simulink model "IEEE_30_Bus_System"  (R2021a)
settings: Solver=FixedStepDiscrete  StartTime=0.0  StopTime=0.5  FixedStep=50e-6  RelTol=1e-3
undefined symbols (not defined in the file): Angle, Magnitude, V_890, Vnom1
libraries: spsThreePhasePISectionLineLib x37, spsThreePhaseVIMeasurementLib x30, spsLoadFlowBusLib x30, spsThreePhaseSeriesRLCLoadLib x21, spsThreePhaseSourceLib x6, spsThreePhaseTransformerTwoWindingsLib x4, spspowerguiLib x1
(part 1 of 2)
settings Model: Creator=liyifu  LastModifiedBy=shiyu
settings SolverCC: AlgebraicLoopSolver=TrustRegion
settings DataIOCC: ReturnWorkspaceOutputs=off
settings DebuggingCC: SFMachineParentedDataDiag=warning  ArithmeticOperatorsInVariantConditions=warning
settings SFSimCC: SimUseLocalCustomCode=off  CustomCodeUndefinedFunction=UseInterfaceOnly
settings RTWCC: RTWUseLocalCustomCode=off

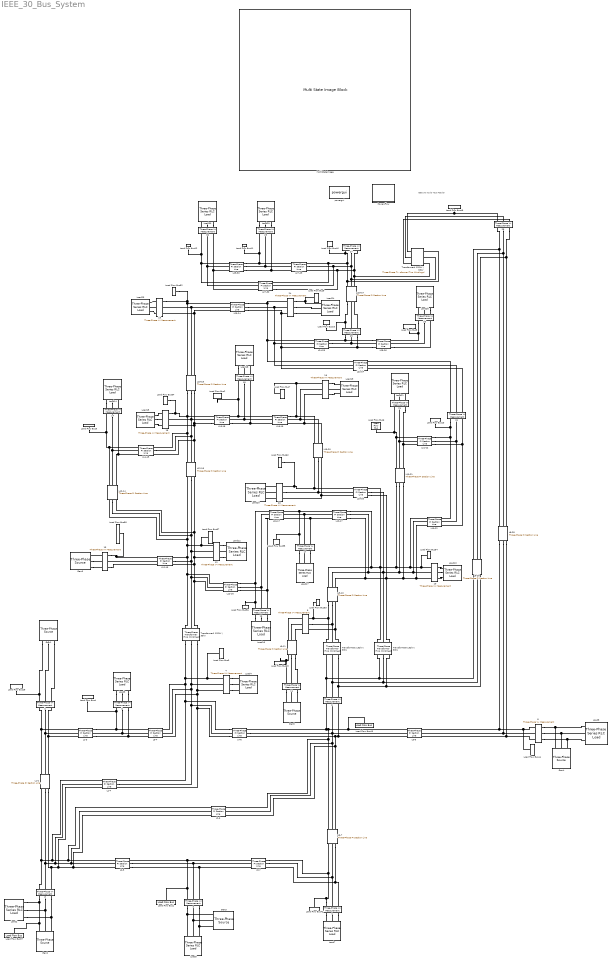
== system IEEE_30_Bus_System ==
  note: IEEE 30 Node Test Feeder
  1 : spsThreePhaseVIMeasurementLib/Three-Phase V-I Measurement  VoltageMeasurement=phase-to-ground  SetLabelV=on  LabelV=Vabc_1  Vpu=on  VpuLL=off  CurrentMeasurement=yes  SetLabelI=on  LabelI=Iabc_1  Ipu=on  Pbase=100e6  Vbase=132e3  OutputType=Magnitude-Angle  PhasorSimulation=off  PSBequivalent=0
  10 : spsThreePhaseVIMeasurementLib/Three-Phase V-I Measurement  VoltageMeasurement=phase-to-ground  SetLabelV=on  LabelV=Vabc_10  Vpu=on  VpuLL=off  CurrentMeasurement=yes  SetLabelI=on  LabelI=Iabc_10  Ipu=on  Pbase=100e6  Vbase=33e3  OutputType=Magnitude-Angle  PhasorSimulation=off  PSBequivalent=0
  11 : spsThreePhaseVIMeasurementLib/Three-Phase V-I Measurement  VoltageMeasurement=phase-to-ground  SetLabelV=on  LabelV=Vabc_11  Vpu=on  VpuLL=off  CurrentMeasurement=yes  SetLabelI=on  LabelI=Iabc_11  Ipu=on  Pbase=100e6  Vbase=33e3  OutputType=Magnitude-Angle  PhasorSimulation=off  PSBequivalent=0
  12 : spsThreePhaseVIMeasurementLib/Three-Phase V-I Measurement  VoltageMeasurement=phase-to-ground  SetLabelV=on  LabelV=Vabc_12  Vpu=on  VpuLL=off  CurrentMeasurement=yes  SetLabelI=on  LabelI=Iabc_12  Ipu=on  Pbase=100e6  Vbase=33e3  OutputType=Magnitude-Angle  PhasorSimulation=off  PSBequivalent=0
  13 : spsThreePhaseVIMeasurementLib/Three-Phase V-I Measurement  VoltageMeasurement=phase-to-ground  SetLabelV=on  LabelV=Vabc_13  Vpu=on  VpuLL=off  CurrentMeasurement=yes  SetLabelI=on  LabelI=Iabc_13  Ipu=on  Pbase=100e6  Vbase=33e3  OutputType=Magnitude-Angle  PhasorSimulation=off  PSBequivalent=0
  14 : spsThreePhaseVIMeasurementLib/Three-Phase V-I Measurement  VoltageMeasurement=phase-to-ground  SetLabelV=on  LabelV=Vabc_14  Vpu=on  VpuLL=off  CurrentMeasurement=yes  SetLabelI=on  LabelI=Iabc_14  Ipu=on  Pbase=100e6  Vbase=33e3  OutputType=Magnitude-Angle  PhasorSimulation=off  PSBequivalent=0
  15 : spsThreePhaseVIMeasurementLib/Three-Phase V-I Measurement  VoltageMeasurement=phase-to-ground  SetLabelV=on  LabelV=Vabc_15  Vpu=on  VpuLL=off  CurrentMeasurement=yes  SetLabelI=on  LabelI=Iabc_15  Ipu=on  Pbase=100e6  Vbase=33e3  OutputType=Magnitude-Angle  PhasorSimulation=off  PSBequivalent=0
  16 : spsThreePhaseVIMeasurementLib/Three-Phase V-I Measurement  VoltageMeasurement=phase-to-ground  SetLabelV=on  LabelV=Vabc_16  Vpu=on  VpuLL=off  CurrentMeasurement=yes  SetLabelI=on  LabelI=Iabc_16  Ipu=on  Pbase=100e6  Vbase=33e3  OutputType=Magnitude-Angle  PhasorSimulation=off  PSBequivalent=0
  17 : spsThreePhaseVIMeasurementLib/Three-Phase V-I Measurement  VoltageMeasurement=phase-to-ground  SetLabelV=on  LabelV=Vabc_17  Vpu=on  VpuLL=off  CurrentMeasurement=yes  SetLabelI=on  LabelI=Iabc_17  Ipu=on  Pbase=100e6  Vbase=33e3  OutputType=Magnitude-Angle  PhasorSimulation=off  PSBequivalent=0
  18 : spsThreePhaseVIMeasurementLib/Three-Phase V-I Measurement  VoltageMeasurement=phase-to-ground  SetLabelV=on  LabelV=Vabc_18  Vpu=on  VpuLL=off  CurrentMeasurement=yes  SetLabelI=on  LabelI=Iabc_18  Ipu=on  Pbase=100e6  Vbase=33e3  OutputType=Magnitude-Angle  PhasorSimulation=off  PSBequivalent=0
  19 : spsThreePhaseVIMeasurementLib/Three-Phase V-I Measurement  VoltageMeasurement=phase-to-ground  SetLabelV=on  LabelV=Vabc_19  Vpu=on  VpuLL=off  CurrentMeasurement=yes  SetLabelI=on  LabelI=Iabc_19  Ipu=on  Pbase=100e6  Vbase=33e3  OutputType=Magnitude-Angle  PhasorSimulation=off  PSBequivalent=0
  2 : spsThreePhaseVIMeasurementLib/Three-Phase V-I Measurement  VoltageMeasurement=phase-to-ground  SetLabelV=on  LabelV=Vabc_2  Vpu=on  VpuLL=off  CurrentMeasurement=yes  SetLabelI=on  LabelI=Iabc_2  Ipu=on  Pbase=100e6  Vbase=132e3  OutputType=Magnitude-Angle  PhasorSimulation=off  PSBequivalent=0
  20 : spsThreePhaseVIMeasurementLib/Three-Phase V-I Measurement  VoltageMeasurement=phase-to-ground  SetLabelV=on  LabelV=Vabc_20  Vpu=on  VpuLL=off  CurrentMeasurement=yes  SetLabelI=on  LabelI=Iabc_20  Ipu=on  Pbase=100e6  Vbase=33e3  OutputType=Magnitude-Angle  PhasorSimulation=off  PSBequivalent=0
  21 : spsThreePhaseVIMeasurementLib/Three-Phase V-I Measurement  VoltageMeasurement=phase-to-ground  SetLabelV=on  LabelV=Vabc_21  Vpu=on  VpuLL=off  CurrentMeasurement=yes  SetLabelI=on  LabelI=Iabc_21  Ipu=on  Pbase=100e6  Vbase=33e3  OutputType=Magnitude-Angle  PhasorSimulation=off  PSBequivalent=0
  22 : spsThreePhaseVIMeasurementLib/Three-Phase V-I Measurement  VoltageMeasurement=phase-to-ground  SetLabelV=on  LabelV=Vabc_22  Vpu=on  VpuLL=off  CurrentMeasurement=yes  SetLabelI=on  LabelI=Iabc_22  Ipu=on  Pbase=100e6  Vbase=33e3  OutputType=Magnitude-Angle  PhasorSimulation=off  PSBequivalent=0
  23 : spsThreePhaseVIMeasurementLib/Three-Phase V-I Measurement  VoltageMeasurement=phase-to-ground  SetLabelV=on  LabelV=Vabc_23  Vpu=on  VpuLL=off  CurrentMeasurement=yes  SetLabelI=on  LabelI=Iabc_23  Ipu=on  Pbase=100e6  Vbase=33e3  OutputType=Magnitude-Angle  PhasorSimulation=off  PSBequivalent=0
  24 : spsThreePhaseVIMeasurementLib/Three-Phase V-I Measurement  VoltageMeasurement=phase-to-ground  SetLabelV=on  LabelV=Vabc_24  Vpu=on  VpuLL=off  CurrentMeasurement=yes  SetLabelI=on  LabelI=Iabc_24  Ipu=on  Pbase=100e6  Vbase=33e3  OutputType=Magnitude-Angle  PhasorSimulation=off  PSBequivalent=0
  25 : spsThreePhaseVIMeasurementLib/Three-Phase V-I Measurement  VoltageMeasurement=phase-to-ground  SetLabelV=on  LabelV=Vabc_25  Vpu=on  VpuLL=off  CurrentMeasurement=yes  SetLabelI=on  LabelI=Iabc_25  Ipu=on  Pbase=100e6  Vbase=33e3  OutputType=Magnitude-Angle  PhasorSimulation=off  PSBequivalent=0
  26 : spsThreePhaseVIMeasurementLib/Three-Phase V-I Measurement  VoltageMeasurement=phase-to-ground  SetLabelV=on  LabelV=Vabc_26  Vpu=on  VpuLL=off  CurrentMeasurement=yes  SetLabelI=on  LabelI=Iabc_26  Ipu=on  Pbase=100e6  Vbase=33e3  OutputType=Magnitude-Angle  PhasorSimulation=off  PSBequivalent=0
  27 : spsThreePhaseVIMeasurementLib/Three-Phase V-I Measurement  VoltageMeasurement=phase-to-ground  SetLabelV=on  LabelV=Vabc_27  Vpu=off  VpuLL=off  CurrentMeasurement=no  SetLabelI=on  LabelI=Iabc_27  Ipu=on  Pbase=100e6  Vbase=33e3  OutputType=Magnitude-Angle  PhasorSimulation=off  PSBequivalent=0
  28 : spsThreePhaseVIMeasurementLib/Three-Phase V-I Measurement  VoltageMeasurement=phase-to-ground  SetLabelV=on  LabelV=Vabc_28  Vpu=on  VpuLL=off  CurrentMeasurement=yes  SetLabelI=on  LabelI=Iabc_28  Ipu=on  Pbase=100e6  Vbase=132e3  OutputType=Magnitude-Angle  PhasorSimulation=off  PSBequivalent=0
  29 : spsThreePhaseVIMeasurementLib/Three-Phase V-I Measurement  VoltageMeasurement=phase-to-ground  SetLabelV=on  LabelV=Vabc_29  Vpu=on  VpuLL=off  CurrentMeasurement=yes  SetLabelI=on  LabelI=Iabc_29  Ipu=on  Pbase=100e6  Vbase=33e3  OutputType=Magnitude-Angle  PhasorSimulation=off  PSBequivalent=0
  3 : spsThreePhaseVIMeasurementLib/Three-Phase V-I Measurement  VoltageMeasurement=phase-to-ground  SetLabelV=on  LabelV=Vabc_3  Vpu=on  VpuLL=off  CurrentMeasurement=yes  SetLabelI=on  LabelI=Iabc_3  Ipu=on  Pbase=100e6  Vbase=132e3  OutputType=Magnitude-Angle  PhasorSimulation=off  PSBequivalent=0
  30 : spsThreePhaseVIMeasurementLib/Three-Phase V-I Measurement  VoltageMeasurement=phase-to-ground  SetLabelV=on  LabelV=Vabc_30  Vpu=on  VpuLL=off  CurrentMeasurement=yes  SetLabelI=on  LabelI=Iabc_30  Ipu=on  Pbase=100e6  Vbase=33e3  OutputType=Magnitude-Angle  PhasorSimulation=off  PSBequivalent=0
  4 : spsThreePhaseVIMeasurementLib/Three-Phase V-I Measurement  VoltageMeasurement=phase-to-ground  SetLabelV=on  LabelV=Vabc_4  Vpu=on  VpuLL=off  CurrentMeasurement=yes  SetLabelI=on  LabelI=Iabc_4  Ipu=on  Pbase=100e6  Vbase=132e3  OutputType=Magnitude-Angle  PhasorSimulation=off  PSBequivalent=0
  5 : spsThreePhaseVIMeasurementLib/Three-Phase V-I Measurement  VoltageMeasurement=phase-to-ground  SetLabelV=on  LabelV=Vabc_5  Vpu=on  VpuLL=off  CurrentMeasurement=yes  SetLabelI=on  LabelI=Iabc_5  Ipu=on  Pbase=100e6  Vbase=132e3  OutputType=Magnitude-Angle  PhasorSimulation=off  PSBequivalent=0
  6 : spsThreePhaseVIMeasurementLib/Three-Phase V-I Measurement  VoltageMeasurement=phase-to-ground  SetLabelV=on  LabelV=Vabc_6  Vpu=on  VpuLL=off  CurrentMeasurement=yes  SetLabelI=on  LabelI=Iabc_6  Ipu=on  Pbase=100e6  Vbase=132e3  OutputType=Magnitude-Angle  PhasorSimulation=off  PSBequivalent=0
  7 : spsThreePhaseVIMeasurementLib/Three-Phase V-I Measurement  VoltageMeasurement=phase-to-ground  SetLabelV=on  LabelV=Vabc_7  Vpu=on  VpuLL=off  CurrentMeasurement=yes  SetLabelI=on  LabelI=Iabc_7  Ipu=on  Pbase=100e6  Vbase=132e3  OutputType=Magnitude-Angle  PhasorSimulation=off  PSBequivalent=0
  8 : spsThreePhaseVIMeasurementLib/Three-Phase V-I Measurement  VoltageMeasurement=phase-to-ground  SetLabelV=on  LabelV=Vabc_8  Vpu=on  VpuLL=off  CurrentMeasurement=yes  SetLabelI=on  LabelI=Iabc_8  Ipu=on  Pbase=100e6  Vbase=132e3  OutputType=Magnitude-Angle  PhasorSimulation=off  PSBequivalent=0
  9 : spsThreePhaseVIMeasurementLib/Three-Phase V-I Measurement  VoltageMeasurement=phase-to-ground  SetLabelV=on  LabelV=Vabc_9  Vpu=on  VpuLL=off  CurrentMeasurement=yes  SetLabelI=on  LabelI=Iabc_9  Ipu=on  Pbase=100e6  Vbase=33e3  OutputType=Magnitude-Angle  PhasorSimulation=off  PSBequivalent=0
  Gen1 : spsThreePhaseSourceLib/Three-Phase Source  InternalConnection=Yg  VoltagePhases=off  Voltage=132e3  PhaseAngle=0  Voltage_phases=[132 132 132]*1e3/sqrt(3)  PhaseAngles_phases=[0 -120 +120]  Frequency=60  NonIdealSource=on  SpecifyImpedance=off  Resistance=10  Inductance=0.15  ShortCircuitLevel=Apparent_power_gen1  BaseVoltage=132e3  XRratio=8  BusType=swing  Pref=2.6095  Qref=-0.1679  Prefabc=[10e3, 10e3, 10e3]  Qrefabc=[0, 0, 0]  Qmin=-inf  Qmax=inf
  Gen2 : spsThreePhaseSourceLib/Three-Phase Source  InternalConnection=Yg  VoltagePhases=off  Voltage=132e3  PhaseAngle=0  Voltage_phases=[132 132 132]*1e3/sqrt(3)  PhaseAngles_phases=[0 -120 +120]  Frequency=60  NonIdealSource=on  SpecifyImpedance=off  Resistance=10  Inductance=0.15  ShortCircuitLevel=Apparent_power_gen1  BaseVoltage=132e3  XRratio=8  BusType=PV  Pref=0.4e8  Qref=0.5000  Prefabc=[10e3, 10e3, 10e3]  Qrefabc=[0, 0, 0]  Qmin=-inf  Qmax=inf
  Gen3 : spsThreePhaseSourceLib/Three-Phase Source  InternalConnection=Yg  VoltagePhases=off  Voltage=132e3  PhaseAngle=0  Voltage_phases=[132 132 132]*1e3/sqrt(3)  PhaseAngles_phases=[0 -120 +120]  Frequency=60  NonIdealSource=on  SpecifyImpedance=off  Resistance=10  Inductance=0.15  ShortCircuitLevel=Apparent_power_gen1  BaseVoltage=132e3  XRratio=8  BusType=PV  Pref=0.0000  Qref=0.3685  Prefabc=[10e3, 10e3, 10e3]  Qrefabc=[0, 0, 0]  Qmin=-inf  Qmax=inf
  Gen4 : spsThreePhaseSourceLib/Three-Phase Source  InternalConnection=Yg  VoltagePhases=off  Voltage=132e3  PhaseAngle=0  Voltage_phases=[132 132 132]*1e3/sqrt(3)  PhaseAngles_phases=[0 -120 +120]  Frequency=60  NonIdealSource=on  SpecifyImpedance=off  Resistance=10  Inductance=0.15  ShortCircuitLevel=Apparent_power_gen1  BaseVoltage=132e3  XRratio=8  BusType=PV  Pref=0.0000  Qref=0.3714  Prefabc=[10e3, 10e3, 10e3]  Qrefabc=[0, 0, 0]  Qmin=-inf  Qmax=inf
  Gen5 : spsThreePhaseSourceLib/Three-Phase Source  InternalConnection=Yg  VoltagePhases=off  Voltage=33e3  PhaseAngle=0  Voltage_phases=[33 33 33]*1e3/sqrt(3)  PhaseAngles_phases=[0 -120 +120]  Frequency=60  NonIdealSource=on  SpecifyImpedance=off  Resistance=10  Inductance=0.15  ShortCircuitLevel=Apparent_power_gen1  BaseVoltage=33e3  XRratio=8  BusType=PV  Pref=0.0000  Qref=0.1617  Prefabc=[10e3, 10e3, 10e3]  Qrefabc=[0, 0, 0]  Qmin=-inf  Qmax=inf
  Gen6 : spsThreePhaseSourceLib/Three-Phase Source  InternalConnection=Yg  VoltagePhases=off  Voltage=33e3  PhaseAngle=0  Voltage_phases=[33 33 33]*1e3/sqrt(3)  PhaseAngles_phases=[0 -120 +120]  Frequency=60  NonIdealSource=on  SpecifyImpedance=off  Resistance=10  Inductance=0.15  ShortCircuitLevel=Apparent_power_gen1  BaseVoltage=33e3  XRratio=8  BusType=PV  Pref=0.0000  Qref=0.1062  Prefabc=[10e3, 10e3, 10e3]  Qrefabc=[0, 0, 0]  Qmin=-inf  Qmax=inf
  L1-2 : spsThreePhasePISectionLineLib/Three-Phase PI Section Line  LConnTagsString=a|b|c  RConnTagsString=A|B|C  Length=1  Frequency=60  Resistances=[0.0192 0.048]*174.24  Inductances=[1.5252e-4 3.8131e-4]*174.24  Capacitances=[1.4006e-4 1.4006e-4]/174.24
  L1-3 : spsThreePhasePISectionLineLib/Three-Phase PI Section Line  LConnTagsString=a|b|c  RConnTagsString=A|B|C  Length=1  Frequency=60  Resistances=[0.0452 0.113]*174.24  Inductances=[4.3821e-4 1.0955e-4]*174.24  Capacitances=[1.0823e-4 1.0823e-4]/174.24
  L10-17 : spsThreePhasePISectionLineLib/Three-Phase PI Section Line  LConnTagsString=a|b|c  RConnTagsString=A|B|C  Length=1  Frequency=60  Resistances=[0.0324 0.081]*10.89  Inductances=[2.2414e-4 5.6036e-4]*10.89  Capacitances=[1e-6 1e-6]/10.89
  L10-20 : spsThreePhasePISectionLineLib/Three-Phase PI Section Line  LConnTagsString=a|b|c  RConnTagsString=A|B|C  Length=1  Frequency=60  Resistances=[0.0936 0.234]*10.89  Inductances=[5.5439e-4 1.3860e-3]*10.89  Capacitances=[1e-6 1e-6]/10.89
  L10-21 : spsThreePhasePISectionLineLib/Three-Phase PI Section Line  LConnTagsString=a|b|c  RConnTagsString=A|B|C  Length=1  Frequency=60  Resistances=[0.0348 0.087]*10.89  Inductances=[1.9868e-4 4.9670e-4]*10.89  Capacitances=[1e-6 1e-6]/10.89
  L10-22 : spsThreePhasePISectionLineLib/Three-Phase PI Section Line  LConnTagsString=a|b|c  RConnTagsString=A|B|C  Length=1  Frequency=60  Resistances=[0.0727 0.18175]*10.89  Inductances=[3.9762e-4 9.9406e-4]*10.89  Capacitances=[1e-6 1e-6]/10.89
  L12-13 : spsThreePhasePISectionLineLib/Three-Phase PI Section Line  LConnTagsString=a|b|c  RConnTagsString=A|B|C  Length=1  Frequency=60  Resistances=[0 0]*10.89  Inductances=[3.7136e-4 9.2840e-4]*10.89  Capacitances=[1e-6 1e-6]/10.89
  L12-14 : spsThreePhasePISectionLineLib/Three-Phase PI Section Line  LConnTagsString=a|b|c  RConnTagsString=A|B|C  Length=1  Frequency=60  Resistances=[0.1231 0.30775]*10.89  Inductances=[6.7880e-4 1.6970e-3]*10.89  Capacitances=[1e-6 1e-6]/10.89
  L12-15 : spsThreePhasePISectionLineLib/Three-Phase PI Section Line  LConnTagsString=a|b|c  RConnTagsString=A|B|C  Length=1  Frequency=60  Resistances=[0.0662 0.1655]*10.89  Inductances=[3.4590e-4 8.6474e-4]*10.89  Capacitances=[1e-6 1e-6]/10.89
  L12-16 : spsThreePhasePISectionLineLib/Three-Phase PI Section Line  LConnTagsString=a|b|c  RConnTagsString=A|B|C  Length=1  Frequency=60  Resistances=[0.0945 0.23625]*10.89  Inductances=[5.2707e-4 1.3177e-3]*10.89  Capacitances=[1e-6 1e-6]/10.89
  L14-15 : spsThreePhasePISectionLineLib/Three-Phase PI Section Line  LConnTagsString=a|b|c  RConnTagsString=A|B|C  Length=1  Frequency=60  Resistances=[0.221 0.5525]*10.89  Inductances=[5.2972e-4 1.3243e-3]*10.89  Capacitances=[1e-6 1e-6]/10.89
  L15-18 : spsThreePhasePISectionLineLib/Three-Phase PI Section Line  LConnTagsString=a|b|c  RConnTagsString=A|B|C  Length=1  Frequency=60  Resistances=[0.1073 0.26825]*10.89  Inductances=[5.7959e-4 1.4490e-3]*10.89  Capacitances=[1e-6 1e-6]/10.89
  L15-23 : spsThreePhasePISectionLineLib/Three-Phase PI Section Line  LConnTagsString=a|b|c  RConnTagsString=A|B|C  Length=1  Frequency=60  Resistances=[0.1 0.25]*10.89  Inductances=[5.3582e-4 1.3396e-3]*10.89  Capacitances=[1e-6 1e-6]/10.89
  L16-17 : spsThreePhasePISectionLineLib/Three-Phase PI Section Line  LConnTagsString=a|b|c  RConnTagsString=A|B|C  Length=1  Frequency=60  Resistances=[0.0524 0.131]*10.89  Inductances=[5.1009e-4 1.2752e-3]*10.89  Capacitances=[1e-6 1e-6]/10.89
  L18-19 : spsThreePhasePISectionLineLib/Three-Phase PI Section Line  LConnTagsString=a|b|c  RConnTagsString=A|B|C  Length=1  Frequency=60  Resistances=[0.0639 0.15975]*10.89  Inductances=[3.4271e-4 8.5678e-4]*10.89  Capacitances=[1e-6 1e-6]/10.89
  L19-20 : spsThreePhasePISectionLineLib/Three-Phase PI Section Line  LConnTagsString=a|b|c  RConnTagsString=A|B|C  Length=1  Frequency=60  Resistances=[0.034 0.085]*10.89  Inductances=[1.8038e-4 4.5094e-4]*10.89  Capacitances=[1e-6 1e-6]/10.89
  L2-4 : spsThreePhasePISectionLineLib/Three-Phase PI Section Line  LConnTagsString=a|b|c  RConnTagsString=A|B|C  Length=1  Frequency=60  Resistances=[0.057 0.1425]*174.24  Inductances=[4.6075e-4 1.1519e-3]*174.24  Capacitances=[9.7615e-5 9.7615e-5]/174.24
  L2-5 : spsThreePhasePISectionLineLib/Three-Phase PI Section Line  LConnTagsString=a|b|c  RConnTagsString=A|B|C  Length=1  Frequency=60  Resistances=[0.0472 0.118]*174.24  Inductances=[5.2601e-4 1.3150e-3]*174.24  Capacitances=[1.1088e-4 1.1088e-4]/174.24
  L2-6 : spsThreePhasePISectionLineLib/Three-Phase PI Section Line  LConnTagsString=a|b|c  RConnTagsString=A|B|C  Length=1  Frequency=60  Resistances=[0.0581 0.14525]*174.24  Inductances=[4.6765e-4 1.1691e-3]*174.24  Capacitances=[9.9206e-5 9.9206e-5]/174.24
  L21-22 : spsThreePhasePISectionLineLib/Three-Phase PI Section Line  LConnTagsString=a|b|c  RConnTagsString=A|B|C  Length=1  Frequency=60  Resistances=[0.0116 0.029]*10.89  Inductances=[6.2601e-5 1.5650e-4]*10.89  Capacitances=[1e-6 1e-6]/10.89
  L22-24 : spsThreePhasePISectionLineLib/Three-Phase PI Section Line  LConnTagsString=a|b|c  RConnTagsString=A|B|C  Length=1  Frequency=60  Resistances=[0.115 0.2875]*10.89  Inductances=[4.7481e-4 1.1870e-3]*10.89  Capacitances=[1e-6 1e-6]/10.89
  L23-24 : spsThreePhasePISectionLineLib/Three-Phase PI Section Line  LConnTagsString=a|b|c  RConnTagsString=A|B|C  Length=1  Frequency=60  Resistances=[0.132 0.33]*10.89  Inductances=[7.1620e-4 1.7905e-3]*10.89  Capacitances=[1e-6 1e-6]/10.89
  L24-25 : spsThreePhasePISectionLineLib/Three-Phase PI Section Line  LConnTagsString=a|b|c  RConnTagsString=A|B|C  Length=1  Frequency=60  Resistances=[0.1885 0.47125]*10.89  Inductances=[8.7323e-4 2.1831e-3]*10.89  Capacitances=[1e-6 1e-6]/10.89
  L25-26 : spsThreePhasePISectionLineLib/Three-Phase PI Section Line  LConnTagsString=a|b|c  RConnTagsString=A|B|C  Length=1  Frequency=60  Resistances=[0.2544 0.636]*10.89  Inductances=[1.008e-3 2.5200e-3]*10.89  Capacitances=[1e-6 1e-6]/10.89
  L25-27 : spsThreePhasePISectionLineLib/Three-Phase PI Section Line  LConnTagsString=a|b|c  RConnTagsString=A|B|C  Length=1  Frequency=60  Resistances=[0.1093 0.27325]*10.89  Inductances=[5.5360e-4 1.3840e-3]*10.89  Capacitances=[1e-6 1e-6]/10.89
  L27-29 : spsThreePhasePISectionLineLib/Three-Phase PI Section Line  LConnTagsString=a|b|c  RConnTagsString=A|B|C  Length=1  Frequency=60  Resistances=[0.2198 0.5495]*10.89  Inductances=[1.1016e-3 2.7540e-3]*10.89  Capacitances=[1e-6 1e-6]/10.89
  L27-30 : spsThreePhasePISectionLineLib/Three-Phase PI Section Line  LConnTagsString=a|b|c  RConnTagsString=A|B|C  Length=1  Frequency=60  Resistances=[0.3202 0.8005]*10.89  Inductances=[1.5987e-3 3.9968e-3]*10.89  Capacitances=[1e-6 1e-6]/10.89
  L29-30 : spsThreePhasePISectionLineLib/Three-Phase PI Section Line  LConnTagsString=a|b|c  RConnTagsString=A|B|C  Length=1  Frequency=60  Resistances=[0.2399 0.59975]*10.89  Inductances=[1.2024e-3 3.0060e-3]*10.89  Capacitances=[1e-6 1e-6]/10.89
  L3-4 : spsThreePhasePISectionLineLib/Three-Phase PI Section Line  LConnTagsString=a|b|c  RConnTagsString=A|B|C  Length=1  Frequency=60  Resistances=[0.0132 0.033]*174.24  Inductances=[1.0053e-4 2.5133e-4]*174.24  Capacitances=[2.2282e-5 2.2282e-5]/174.24
  L4-6 : spsThreePhasePISectionLineLib/Three-Phase PI Section Line  LConnTagsString=a|b|c  RConnTagsString=A|B|C  Length=1  Frequency=60  Resistances=[0.0119 0.02975]*174.24  Inductances=[1.0982e-4 2.7452e-4]*174.24  Capacitances=[2.3873e-5 2.3873e-5]/174.24
  L5-7 : spsThreePhasePISectionLineLib/Three-Phase PI Section Line  LConnTagsString=a|b|c  RConnTagsString=A|B|C  Length=1  Frequency=60  Resistances=[0.046 0.115]*174.24  Inductances=[3.0770e-4 7.6925e-4]*174.24  Capacitances=[5.4113e-5 5.4113e-5]/174.24
  L6-28 : spsThreePhasePISectionLineLib/Three-Phase PI Section Line  LConnTagsString=a|b|c  RConnTagsString=A|B|C  Length=1  Frequency=60  Resistances=[0.0169 0.04225]*174.24  Inductances=[1.5889e-4 3.9722e-4]*174.24  Capacitances=[3.4484e-5 3.4484e-5]/174.24
  L6-7 : spsThreePhasePISectionLineLib/Three-Phase PI Section Line  LConnTagsString=a|b|c  RConnTagsString=A|B|C  Length=1  Frequency=60  Resistances=[0.0267 0.06675]*174.24  Inductances=[2.1751e-4 5.4378e-4]*174.24  Capacitances=[4.5094e-5 4.5094e-5]/174.24
  L6-8 : spsThreePhasePISectionLineLib/Three-Phase PI Section Line  LConnTagsString=a|b|c  RConnTagsString=A|B|C  Length=1  Frequency=60  Resistances=[0.012 0.03]*174.24  Inductances=[1.1141e-4 2.7852e-4]*174.24  Capacitances=[2.3873e-5 2.3873e-5]/174.24
  L8-28 : spsThreePhasePISectionLineLib/Three-Phase PI Section Line  LConnTagsString=a|b|c  RConnTagsString=A|B|C  Length=1  Frequency=60  Resistances=[0.0636 0.159]*174.24  Inductances=[5.3052e-4 1.3263e-3]*174.24  Capacitances=[1.1353e-4 1.1353e-4]/174.24
  L9-10 : spsThreePhasePISectionLineLib/Three-Phase PI Section Line  LConnTagsString=a|b|c  RConnTagsString=A|B|C  Length=1  Frequency=60  Resistances=[0 0]*10.89  Inductances=[2.9178e-4 7.2946e-4]*10.89  Capacitances=[1e-6 1e-6]/10.89
  L9-11 : spsThreePhasePISectionLineLib/Three-Phase PI Section Line  LConnTagsString=a|b|c  RConnTagsString=A|B|C  Length=1  Frequency=60  Resistances=[0 0]*10.89  Inductances=[5.5174e-4 1.3793e-3]*10.89  Capacitances=[1e-6 1e-6]/10.89
  Load Flow Bus1 : spsLoadFlowBusLib/Load Flow Bus  LConnTagsString=a  Phases=single  Connectors=on both sides  ID=BUS5  Vbase=132e3  Vref=1  Vangle=0  VLF=1  VLFb=1  VLFc=1  angleLF=0  angleLFb=0  angleLFc=0
      settings: AttributesFormatString=%<ID>  SourceProductBaseCode=PS
  Load Flow Bus10 : spsLoadFlowBusLib/Load Flow Bus  LConnTagsString=a  Phases=single  Connectors=on both sides  ID=BUS25  Vbase=33e3  Vref=1  Vangle=0  VLF=1  VLFb=1  VLFc=1  angleLF=0  angleLFb=0  angleLFc=0
      settings: AttributesFormatString=%<ID>  SourceProductBaseCode=PS
  Load Flow Bus11 : spsLoadFlowBusLib/Load Flow Bus  LConnTagsString=a  Phases=single  Connectors=on both sides  ID=BUS29  Vbase=33e3  Vref=1  Vangle=0  VLF=1  VLFb=1  VLFc=1  angleLF=0  angleLFb=0  angleLFc=0
      settings: AttributesFormatString=%<ID>  SourceProductBaseCode=PS
  Load Flow Bus12 : spsLoadFlowBusLib/Load Flow Bus  LConnTagsString=a  Phases=single  Connectors=on both sides  ID=BUS30  Vbase=33e3  Vref=1  Vangle=0  VLF=1  VLFb=1  VLFc=1  angleLF=0  angleLFb=0  angleLFc=0
      settings: AttributesFormatString=%<ID>  SourceProductBaseCode=PS
  Load Flow Bus13 : spsLoadFlowBusLib/Load Flow Bus  LConnTagsString=a  Phases=single  Connectors=on both sides  ID=BUS22  Vbase=33e3  Vref=1  Vangle=0  VLF=1  VLFb=1  VLFc=1  angleLF=0  angleLFb=0  angleLFc=0
      settings: AttributesFormatString=%<ID>  SourceProductBaseCode=PS
  Load Flow Bus2 : spsLoadFlowBusLib/Load Flow Bus  LConnTagsString=a  Phases=single  Connectors=on both sides  ID=BUS18  Vbase=33e3  Vref=1  Vangle=0  VLF=1  VLFb=1  VLFc=1  angleLF=0  angleLFb=0  angleLFc=0
      settings: AttributesFormatString=%<ID>  SourceProductBaseCode=PS
  Load Flow Bus28 : spsLoadFlowBusLib/Load Flow Bus  LConnTagsString=a  Phases=single  Connectors=on both sides  ID=BUS1  Vbase=132e3  Vref=1  Vangle=0  VLF=1  VLFb=1  VLFc=1  angleLF=0  angleLFb=0  angleLFc=0
      settings: AttributesFormatString=%<ID>  SourceProductBaseCode=PS
  Load Flow Bus3 : spsLoadFlowBusLib/Load Flow Bus  LConnTagsString=a  Phases=single  Connectors=on both sides  ID=BUS4  Vbase=132e3  Vref=1  Vangle=0  VLF=1  VLFb=1  VLFc=1  angleLF=0  angleLFb=0  angleLFc=0
      settings: AttributesFormatString=%<ID>  SourceProductBaseCode=PS
  Load Flow Bus37 : spsLoadFlowBusLib/Load Flow Bus  LConnTagsString=a  Phases=single  Connectors=on both sides  ID=BUS2  Vbase=132e3  Vref=1  Vangle=0  VLF=1  VLFb=1  VLFc=1  angleLF=0  angleLFb=0  angleLFc=0
      settings: AttributesFormatString=%<ID>  SourceProductBaseCode=PS
  Load Flow Bus4 : spsLoadFlowBusLib/Load Flow Bus  LConnTagsString=a  Phases=single  Connectors=on both sides  ID=BUS3  Vbase=132e3  Vref=1  Vangle=0  VLF=1  VLFb=1  VLFc=1  angleLF=0  angleLFb=0  angleLFc=0
      settings: AttributesFormatString=%<ID>  SourceProductBaseCode=PS
  Load Flow Bus42 : spsLoadFlowBusLib/Load Flow Bus  LConnTagsString=a  Phases=single  Connectors=on one side  ID=BUS7  Vbase=132e3  Vref=1  Vangle=0  VLF=1  VLFb=1  VLFc=1  angleLF=0  angleLFb=0  angleLFc=0
      settings: AttributesFormatString=%<ID>  SourceProductBaseCode=PS
  Load Flow Bus43 : spsLoadFlowBusLib/Load Flow Bus  LConnTagsString=a  Phases=single  Connectors=on both sides  ID=BUS6  Vbase=132e3  Vref=1  Vangle=0  VLF=1  VLFb=1  VLFc=1  angleLF=0  angleLFb=0  angleLFc=0
      settings: AttributesFormatString=%<ID>  SourceProductBaseCode=PS
  Load Flow Bus44 : spsLoadFlowBusLib/Load Flow Bus  LConnTagsString=a  Phases=single  Connectors=on both sides  ID=BUS8  Vbase=132e3  Vref=1  Vangle=0  VLF=1  VLFb=1  VLFc=1  angleLF=0  angleLFb=0  angleLFc=0
      settings: AttributesFormatString=%<ID>  SourceProductBaseCode=PS
  Load Flow Bus45 : spsLoadFlowBusLib/Load Flow Bus  LConnTagsString=a  Phases=single  Connectors=on one side  ID=BUS28  Vbase=132e3  Vref=1  Vangle=0  VLF=1  VLFb=1  VLFc=1  angleLF=0  angleLFb=0  angleLFc=0
      settings: AttributesFormatString=%<ID>  SourceProductBaseCode=PS
  Load Flow Bus46 : spsLoadFlowBusLib/Load Flow Bus  LConnTagsString=a  Phases=single  Connectors=on one side  ID=BUS27  Vbase=33e3  Vref=1  Vangle=0  VLF=1  VLFb=1  VLFc=1  angleLF=0  angleLFb=0  angleLFc=0
      settings: AttributesFormatString=%<ID>  SourceProductBaseCode=PS
  Load Flow Bus5 : spsLoadFlowBusLib/Load Flow Bus  LConnTagsString=a  Phases=single  Connectors=on both sides  ID=BUS14  Vbase=33e3  Vref=1  Vangle=0  VLF=1  VLFb=1  VLFc=1  angleLF=0  angleLFb=0  angleLFc=0
      settings: AttributesFormatString=%<ID>  SourceProductBaseCode=PS
  Load Flow Bus52 : spsLoadFlowBusLib/Load Flow Bus  LConnTagsString=a  Phases=single  Connectors=on both sides  ID=BUS23  Vbase=33e3  Vref=1  Vangle=0  VLF=1  VLFb=1  VLFc=1  angleLF=0  angleLFb=0  angleLFc=0
      settings: AttributesFormatString=%<ID>  SourceProductBaseCode=PS
  Load Flow Bus53 : spsLoadFlowBusLib/Load Flow Bus  LConnTagsString=a  Phases=single  Connectors=on both sides  ID=BUS9  Vbase=33e3  Vref=1  Vangle=0  VLF=1  VLFb=1  VLFc=1  angleLF=0  angleLFb=0  angleLFc=0
      settings: AttributesFormatString=%<ID>  SourceProductBaseCode=PS
  Load Flow Bus54 : spsLoadFlowBusLib/Load Flow Bus  LConnTagsString=a  Phases=single  Connectors=on both sides  ID=BUS10  Vbase=33e3  Vref=1  Vangle=0  VLF=1  VLFb=1  VLFc=1  angleLF=0  angleLFb=0  angleLFc=0
      settings: AttributesFormatString=%<ID>  SourceProductBaseCode=PS
  Load Flow Bus55 : spsLoadFlowBusLib/Load Flow Bus  LConnTagsString=a  Phases=single  Connectors=on both sides  ID=BUS17  Vbase=33e3  Vref=1  Vangle=0  VLF=1  VLFb=1  VLFc=1  angleLF=0  angleLFb=0  angleLFc=0
      settings: AttributesFormatString=%<ID>  SourceProductBaseCode=PS
  Load Flow Bus56 : spsLoadFlowBusLib/Load Flow Bus  LConnTagsString=a  Phases=single  Connectors=on both sides  ID=BUS16  Vbase=33e3  Vref=1  Vangle=0  VLF=1  VLFb=1  VLFc=1  angleLF=0  angleLFb=0  angleLFc=0
      settings: AttributesFormatString=%<ID>  SourceProductBaseCode=PS
  Load Flow Bus57 : spsLoadFlowBusLib/Load Flow Bus  LConnTagsString=a  Phases=single  Connectors=on both sides  ID=BUS12  Vbase=33e3  Vref=1  Vangle=0  VLF=1  VLFb=1  VLFc=1  angleLF=0  angleLFb=0  angleLFc=0
      settings: AttributesFormatString=%<ID>  SourceProductBaseCode=PS
  Load Flow Bus58 : spsLoadFlowBusLib/Load Flow Bus  LConnTagsString=a  Phases=single  Connectors=on both sides  ID=BUS13  Vbase=33e3  Vref=1  Vangle=0  VLF=1  VLFb=1  VLFc=1  angleLF=0  angleLFb=0  angleLFc=0
      settings: AttributesFormatString=%<ID>  SourceProductBaseCode=PS
  Load Flow Bus6 : spsLoadFlowBusLib/Load Flow Bus  LConnTagsString=a  Phases=single  Connectors=on both sides  ID=BUS21  Vbase=33e3  Vref=1  Vangle=0  VLF=1  VLFb=1  VLFc=1  angleLF=0  angleLFb=0  angleLFc=0
      settings: AttributesFormatString=%<ID>  SourceProductBaseCode=PS
  Load Flow Bus62 : spsLoadFlowBusLib/Load Flow Bus  LConnTagsString=a  Phases=single  Connectors=on both sides  ID=BUS20  Vbase=33e3  Vref=1  Vangle=0  VLF=1  VLFb=1  VLFc=1  angleLF=0  angleLFb=0  angleLFc=0
      settings: AttributesFormatString=%<ID>  SourceProductBaseCode=PS
  Load Flow Bus63 : spsLoadFlowBusLib/Load Flow Bus  LConnTagsString=a  Phases=single  Connectors=on both sides  ID=BUS11  Vbase=33e3  Vref=1  Vangle=0  VLF=1  VLFb=1  VLFc=1  angleLF=0  angleLFb=0  angleLFc=0
      settings: AttributesFormatString=%<ID>  SourceProductBaseCode=PS
  Load Flow Bus64 : spsLoadFlowBusLib/Load Flow Bus  LConnTagsString=a  Phases=single  Connectors=on both sides  ID=BUS15  Vbase=33e3  Vref=1  Vangle=0  VLF=1  VLFb=1  VLFc=1  angleLF=0  angleLFb=0  angleLFc=0
      settings: AttributesFormatString=%<ID>  SourceProductBaseCode=PS
  Load Flow Bus7 : spsLoadFlowBusLib/Load Flow Bus  LConnTagsString=a  Phases=single  Connectors=on both sides  ID=BUS19  Vbase=33e3  Vref=1  Vangle=0  VLF=1  VLFb=1  VLFc=1  angleLF=0  angleLFb=0  angleLFc=0
      settings: AttributesFormatString=%<ID>  SourceProductBaseCode=PS
  Load Flow Bus8 : spsLoadFlowBusLib/Load Flow Bus  LConnTagsString=a  Phases=single  Connectors=on both sides  ID=BUS26  Vbase=33e3  Vref=1  Vangle=0  VLF=1  VLFb=1  VLFc=1  angleLF=0  angleLFb=0  angleLFc=0
      settings: AttributesFormatString=%<ID>  SourceProductBaseCode=PS
  Load Flow Bus9 : spsLoadFlowBusLib/Load Flow Bus  LConnTagsString=a  Phases=single  Connectors=on both sides  ID=BUS24  Vbase=33e3  Vref=1  Vangle=0  VLF=1  VLFb=1  VLFc=1  angleLF=0  angleLFb=0  angleLFc=0
      settings: AttributesFormatString=%<ID>  SourceProductBaseCode=PS
  Load10 : spsThreePhaseSeriesRLCLoadLib/Three-Phase Series RLC Load  LConnTagsString=A|B|C  Configuration=Y (grounded)  NominalVoltage=33e3  Vabc=[1e3 1e3 1e3]  Vabcp=V_890*Vnom1  NominalFrequency=60  UnbalancedPower=off  ActivePower=1.93333e6  InductivePower=0.66667e6  CapacitivePower=0  Pabc=[10e3 9e3 11e3]  QLabc=[100 90 110]  QCabc=[100 90 110]  Pabcp=Pa_890  QLabcp=Pp_890  QCabcp=Pn_890  Measurements=None  LoadType=constant PQ
  Load12 : spsThreePhaseSeriesRLCLoadLib/Three-Phase Series RLC Load  LConnTagsString=A|B|C  Configuration=Y (grounded)  NominalVoltage=33e3  Vabc=[1e3 1e3 1e3]  Vabcp=V_890*Vnom1  NominalFrequency=60  UnbalancedPower=off  ActivePower=3.73333e6  InductivePower=2.5e6  CapacitivePower=0  Pabc=[10e3 9e3 11e3]  QLabc=[100 90 110]  QCabc=[100 90 110]  Pabcp=Pa_890  QLabcp=Pp_890  QCabcp=Pn_890  Measurements=None  LoadType=constant PQ
  Load14 : spsThreePhaseSeriesRLCLoadLib/Three-Phase Series RLC Load  LConnTagsString=A|B|C  Configuration=Y (grounded)  NominalVoltage=33e3  Vabc=[1e3 1e3 1e3]  Vabcp=V_890*Vnom1  NominalFrequency=60  UnbalancedPower=off  ActivePower=2.06667e6  InductivePower=0.53333e6  CapacitivePower=0  Pabc=[10e3 9e3 11e3]  QLabc=[100 90 110]  QCabc=[100 90 110]  Pabcp=Pa_890  QLabcp=Pp_890  QCabcp=Pn_890  Measurements=None  LoadType=constant PQ
  Load15 : spsThreePhaseSeriesRLCLoadLib/Three-Phase Series RLC Load  LConnTagsString=A|B|C  Configuration=Y (grounded)  NominalVoltage=33e3  Vabc=[1e3 1e3 1e3]  Vabcp=V_890*Vnom1  NominalFrequency=60  UnbalancedPower=off  ActivePower=2.73333e6  InductivePower=0.833333e6  CapacitivePower=0  Pabc=[10e3 9e3 11e3]  QLabc=[100 90 110]  QCabc=[100 90 110]  Pabcp=Pa_890  QLabcp=Pp_890  QCabcp=Pn_890  Measurements=None  LoadType=constant PQ
  Load16 : spsThreePhaseSeriesRLCLoadLib/Three-Phase Series RLC Load  LConnTagsString=A|B|C  Configuration=Y (grounded)  NominalVoltage=33e3  Vabc=[1e3 1e3 1e3]  Vabcp=V_890*Vnom1  NominalFrequency=60  UnbalancedPower=off  ActivePower=1.166667e6  InductivePower=0.6e6  CapacitivePower=0  Pabc=[10e3 9e3 11e3]  QLabc=[100 90 110]  QCabc=[100 90 110]  Pabcp=Pa_890  QLabcp=Pp_890  QCabcp=Pn_890  Measurements=None  LoadType=constant PQ
  Load17 : spsThreePhaseSeriesRLCLoadLib/Three-Phase Series RLC Load  LConnTagsString=A|B|C  Configuration=Y (grounded)  NominalVoltage=33e3  Vabc=[1e3 1e3 1e3]  Vabcp=V_890*Vnom1  NominalFrequency=60  UnbalancedPower=off  ActivePower=3.0e6  InductivePower=1.93333e6  CapacitivePower=0  Pabc=[10e3 9e3 11e3]  QLabc=[100 90 110]  QCabc=[100 90 110]  Pabcp=Pa_890  QLabcp=Pp_890  QCabcp=Pn_890  Measurements=None  LoadType=constant PQ
  Load18 : spsThreePhaseSeriesRLCLoadLib/Three-Phase Series RLC Load  LConnTagsString=A|B|C  Configuration=Y (grounded)  NominalVoltage=33e3  Vabc=[1e3 1e3 1e3]  Vabcp=V_890*Vnom1  NominalFrequency=60  UnbalancedPower=off  ActivePower=1.06667e6  InductivePower=0.3e6  CapacitivePower=0  Pabc=[10e3 9e3 11e3]  QLabc=[100 90 110]  QCabc=[100 90 110]  Pabcp=Pa_890  QLabcp=Pp_890  QCabcp=Pn_890  Measurements=None  LoadType=constant PQ
  Load19 : spsThreePhaseSeriesRLCLoadLib/Three-Phase Series RLC Load  LConnTagsString=A|B|C  Configuration=Y (grounded)  NominalVoltage=33e3  Vabc=[1e3 1e3 1e3]  Vabcp=V_890*Vnom1  NominalFrequency=60  UnbalancedPower=off  ActivePower=3.16667e6  InductivePower=1.133333e6  CapacitivePower=0  Pabc=[10e3 9e3 11e3]  QLabc=[100 90 110]  QCabc=[100 90 110]  Pabcp=Pa_890  QLabcp=Pp_890  QCabcp=Pn_890  Measurements=None  LoadType=constant PQ
  Load2 : spsThreePhaseSeriesRLCLoadLib/Three-Phase Series RLC Load  LConnTagsString=A|B|C  Configuration=Y (grounded)  NominalVoltage=132e3  Vabc=[1e3 1e3 1e3]  Vabcp=V_890*Vnom1  NominalFrequency=60  UnbalancedPower=off  ActivePower=7.23333e6  InductivePower=4.23333e6  CapacitivePower=0  Pabc=[10e3 9e3 11e3]  QLabc=[100 90 110]  QCabc=[100 90 110]  Pabcp=Pa_890  QLabcp=Pp_890  QCabcp=Pn_890  Measurements=None  LoadType=constant PQ
  Load20 : spsThreePhaseSeriesRLCLoadLib/Three-Phase Series RLC Load  LConnTagsString=A|B|C  Configuration=Y (grounded)  NominalVoltage=33e3  Vabc=[1e3 1e3 1e3]  Vabcp=V_890*Vnom1  NominalFrequency=60  UnbalancedPower=off  ActivePower=0.73333e6  InductivePower=0.233333e6  CapacitivePower=0  Pabc=[10e3 9e3 11e3]  QLabc=[100 90 110]  QCabc=[100 90 110]  Pabcp=Pa_890  QLabcp=Pp_890  QCabcp=Pn_890  Measurements=None  LoadType=constant PQ
  Load21 : spsThreePhaseSeriesRLCLoadLib/Three-Phase Series RLC Load  LConnTagsString=A|B|C  Configuration=Y (grounded)  NominalVoltage=33e3  Vabc=[1e3 1e3 1e3]  Vabcp=V_890*Vnom1  NominalFrequency=60  UnbalancedPower=off  ActivePower=5.83333e6  InductivePower=3.73333e6  CapacitivePower=0  Pabc=[10e3 9e3 11e3]  QLabc=[100 90 110]  QCabc=[100 90 110]  Pabcp=Pa_890  QLabcp=Pp_890  QCabcp=Pn_890  Measurements=None  LoadType=constant PQ
  Load23 : spsThreePhaseSeriesRLCLoadLib/Three-Phase Series RLC Load  LConnTagsString=A|B|C  Configuration=Y (grounded)  NominalVoltage=33e3  Vabc=[1e3 1e3 1e3]  Vabcp=V_890*Vnom1  NominalFrequency=60  UnbalancedPower=off  ActivePower=1.06667e6  InductivePower=0.53333e6  CapacitivePower=0  Pabc=[10e3 9e3 11e3]  QLabc=[100 90 110]  QCabc=[100 90 110]  Pabcp=Pa_890  QLabcp=Pp_890  QCabcp=Pn_890  Measurements=None  LoadType=constant PQ
  Load24 : spsThreePhaseSeriesRLCLoadLib/Three-Phase Series RLC Load  LConnTagsString=A|B|C  Configuration=Y (grounded)  NominalVoltage=33e3  Vabc=[1e3 1e3 1e3]  Vabcp=V_890*Vnom1  NominalFrequency=60  UnbalancedPower=off  ActivePower=2.9e6  InductivePower=2.23333e6  CapacitivePower=0  Pabc=[10e3 9e3 11e3]  QLabc=[100 90 110]  QCabc=[100 90 110]  Pabcp=Pa_890  QLabcp=Pp_890  QCabcp=Pn_890  Measurements=None  LoadType=constant PQ
  Load26 : spsThreePhaseSeriesRLCLoadLib/Three-Phase Series RLC Load  LConnTagsString=A|B|C  Configuration=Y (grounded)  NominalVoltage=33e3  Vabc=[1e3 1e3 1e3]  Vabcp=V_890*Vnom1  NominalFrequency=60  UnbalancedPower=off  ActivePower=1.16667e6  InductivePower=0.76667e6  CapacitivePower=0  Pabc=[10e3 9e3 11e3]  QLabc=[100 90 110]  QCabc=[100 90 110]  Pabcp=Pa_890  QLabcp=Pp_890  QCabcp=Pn_890  Measurements=None  LoadType=constant PQ
  Load29 : spsThreePhaseSeriesRLCLoadLib/Three-Phase Series RLC Load  LConnTagsString=A|B|C  Configuration=Y (grounded)  NominalVoltage=33e3  Vabc=[1e3 1e3 1e3]  Vabcp=V_890*Vnom1  NominalFrequency=60  UnbalancedPower=off  ActivePower=0.8e6  InductivePower=0.3e6  CapacitivePower=0  Pabc=[10e3 9e3 11e3]  QLabc=[100 90 110]  QCabc=[100 90 110]  Pabcp=Pa_890  QLabcp=Pp_890  QCabcp=Pn_890  Measurements=None  LoadType=constant PQ
  Load3 : spsThreePhaseSeriesRLCLoadLib/Three-Phase Series RLC Load  LConnTagsString=A|B|C  Configuration=Y (grounded)  NominalVoltage=132e3  Vabc=[1e3 1e3 1e3]  Vabcp=V_890*Vnom1  NominalFrequency=60  UnbalancedPower=off  ActivePower=0.8e6  InductivePower=0.4e6  CapacitivePower=0  Pabc=[10e3 9e3 11e3]  QLabc=[100 90 110]  QCabc=[100 90 110]  Pabcp=Pa_890  QLabcp=Pp_890  QCabcp=Pn_890  Measurements=None  LoadType=constant PQ
  Load30 : spsThreePhaseSeriesRLCLoadLib/Three-Phase Series RLC Load  LConnTagsString=A|B|C  Configuration=Y (grounded)  NominalVoltage=33e3  Vabc=[1e3 1e3 1e3]  Vabcp=V_890*Vnom1  NominalFrequency=60  UnbalancedPower=off  ActivePower=3.53333e6  InductivePower=0.633333e6  CapacitivePower=0  Pabc=[10e3 9e3 11e3]  QLabc=[100 90 110]  QCabc=[100 90 110]  Pabcp=Pa_890  QLabcp=Pp_890  QCabcp=Pn_890  Measurements=None  LoadType=constant PQ
  Load4 : spsThreePhaseSeriesRLCLoadLib/Three-Phase Series RLC Load  LConnTagsString=A|B|C  Configuration=Y (grounded)  NominalVoltage=132e3  Vabc=[1e3 1e3 1e3]  Vabcp=V_890*Vnom1  NominalFrequency=60  UnbalancedPower=off  ActivePower=2.53333e6  InductivePower=0.53333e6  CapacitivePower=0  Pabc=[10e3 9e3 11e3]  QLabc=[100 90 110]  QCabc=[100 90 110]  Pabcp=Pa_890  QLabcp=Pp_890  QCabcp=Pn_890  Measurements=None  LoadType=constant PQ
  Load5 : spsThreePhaseSeriesRLCLoadLib/Three-Phase Series RLC Load  LConnTagsString=A|B|C  Configuration=Y (grounded)  NominalVoltage=132e3  Vabc=[1e3 1e3 1e3]  Vabcp=V_890*Vnom1  NominalFrequency=60  UnbalancedPower=off  ActivePower=31.4e6  InductivePower=6.3333e6  CapacitivePower=0  Pabc=[10e3 9e3 11e3]  QLabc=[100 90 110]  QCabc=[100 90 110]  Pabcp=Pa_890  QLabcp=Pp_890  QCabcp=Pn_890  Measurements=None  LoadType=constant PQ
  Load7 : spsThreePhaseSeriesRLCLoadLib/Three-Phase Series RLC Load  LConnTagsString=A|B|C  Configuration=Y (grounded)  NominalVoltage=132e3  Vabc=[1e3 1e3 1e3]  Vabcp=V_890*Vnom1  NominalFrequency=60  UnbalancedPower=off  ActivePower=7.6e6  InductivePower=6.63333e6  CapacitivePower=0  Pabc=[10e3 9e3 11e3]  QLabc=[100 90 110]  QCabc=[100 90 110]  Pabcp=Pa_890  QLabcp=Pp_890  QCabcp=Pn_890  Measurements=None  LoadType=constant PQ
  Load8 : spsThreePhaseSeriesRLCLoadLib/Three-Phase Series RLC Load  LConnTagsString=A|B|C  Configuration=Y (grounded)  NominalVoltage=132e3  Vabc=[1e3 1e3 1e3]  Vabcp=V_890*Vnom1  NominalFrequency=60  UnbalancedPower=off  ActivePower=10.0e6  InductivePower=10.0e6  CapacitivePower=0  Pabc=[10e3 9e3 11e3]  QLabc=[100 90 110]  QCabc=[100 90 110]  Pabcp=Pa_890  QLabcp=Pp_890  QCabcp=Pn_890  Measurements=None  LoadType=constant PQ
  MultiStateImage : MultiStateImageBlock  LabelPosition=Bottom
  Power-Flow : Subsystem
      mask Display: disp('Power-Flow\nResults')
  Transformer1 132kV / 33kV : spsThreePhaseTransformerTwoWindingsLib/Three-Phase Transformer (Two Windings)  Winding1Connection=Yg  Winding2Connection=Yg  CoreType=Three single-phase transformers  SetSaturation=off  Hysteresis=off  DataFile='hysteresis'  SetInitialFlux=off  Measurements=None  UNITS=pu  NominalPower=[100e6, 60]  Winding1=[132e3, 0, 6.7906e-4]  Winding2=[33e3, 0, 6.7906e-4]  Rm=2000  Lm=1000  L0=0.5  Saturation=[ 0,0 ; 0.0024,1.2 ; 1.0,1.52 ]  InitialFluxes=[ 0.8 , -0.8 , 0.7 ]  BreakLoop=off  DiscreteSolver=Trapezoidal iterative  DataType=off  TransfoNumber=1
  Transformer2 132kV / 33kV : spsThreePhaseTransformerTwoWindingsLib/Three-Phase Transformer (Two Windings)  Winding1Connection=Yg  Winding2Connection=Yg  CoreType=Three single-phase transformers  SetSaturation=off  Hysteresis=off  DataFile='hysteresis'  SetInitialFlux=off  Measurements=None  UNITS=pu  NominalPower=[100e6, 60]  Winding1=[132e3, 0, 5.5174e-4]  Winding2=[33e3, 0, 5.5174e-4]  Rm=2000  Lm=1000  L0=0.5  Saturation=[ 0,0 ; 0.0024,1.2 ; 1.0,1.52 ]  InitialFluxes=[ 0.8 , -0.8 , 0.7 ]  BreakLoop=off  DiscreteSolver=Trapezoidal iterative  DataType=off  TransfoNumber=1
  Transformer3 132kV / 33kV : spsThreePhaseTransformerTwoWindingsLib/Three-Phase Transformer (Two Windings)  Winding1Connection=Yg  Winding2Connection=Yg  CoreType=Three single-phase transformers  SetSaturation=off  Hysteresis=off  DataFile='hysteresis'  SetInitialFlux=off  Measurements=None  UNITS=pu  NominalPower=[ 100e6 , 60 ]  Winding1=[ 132e3 , 0 , 1.4748e-3 ]  Winding2=[ 33e3 , 0 , 1.4748e-3 ]  Rm=2000  Lm=1000  L0=0.5  Saturation=[ 0,0 ; 0.0024,1.2 ; 1.0,1.52 ]  InitialFluxes=[ 0.8 , -0.8 , 0.7 ]  BreakLoop=off  DiscreteSolver=Trapezoidal iterative  DataType=off  TransfoNumber=1
  Transformer4 132kV / 33kV : spsThreePhaseTransformerTwoWindingsLib/Three-Phase Transformer (Two Windings)  Winding1Connection=Yg  Winding2Connection=Yg  CoreType=Three single-phase transformers  SetSaturation=off  Hysteresis=off  DataFile='hysteresis'  SetInitialFlux=off  Measurements=None  UNITS=pu  NominalPower=[ 100e6 , 60 ]  Winding1=[ 132e3 , 0 , 1.0504e-3 ]  Winding2=[ 33e3 , 0 , 1.0504e-3 ]  Rm=2000  Lm=1000  L0=0.5  Saturation=[ 0,0 ; 0.0024,1.2 ; 1.0,1.52 ]  InitialFluxes=[ 0.8 , -0.8 , 0.7 ]  BreakLoop=off  DiscreteSolver=Trapezoidal iterative  DataType=off  TransfoNumber=1
  powergui : spspowerguiLib/powergui  Priority=1  SimulationMode=Discrete  SampleTime=50e-6  frequency=60  Iterations=50  frequencyindice=60  Pbase=100e3  ErrMax=0.0001  UnitsV=kV  UnitsW=kW  buscounter=0  FunctionMessages=off  echomessages=off  EnableUseOfTLC=off  CurrentSourceSwitches=off  DisableSnubberDevices=off  DisableRonSwitches=off  DisableVfSwitches=off  DisplayEquations=off  AutomaticDiscreteSolvers=off  SolverType=Tustin/Backward Euler (TBE)  Interpol=off  ExternalGateDelay=off  methode=off  Ts=100  x0status=blocks  SPID=off  SwTol=0  HookPort=off  NonlinearTolerance=1e-4  nMaxIteration=100  ContinueOnMaxIteration=off  RestoreLinks=warning  ResistiveCurrentMeasurement=off  Frange=[0:2:500]  Ylog=off  Xlog=on  ShowGrid=off  save=off  variable=ZData  structure=logsout  ZoomFFT=on  StartTime=0.0  cycles=1  DisplayStyle=1  fundamental=60  FreqAxis=off  MaxFrequency=1000  frequencyindicesteady=1  RmsSteady=1  display=off
  connections:
  Load Flow Bus46/LConn1 -- 27/RConn1 -- L25-27/RConn1 -- Transformer4 132kV / 33kV/RConn1 -- L27-29/RConn1 -- L27-30/RConn1
  L25-27/RConn2 -- Transformer4 132kV / 33kV/RConn2 -- 27/RConn2 -- L27-29/RConn2 -- L27-30/RConn2
  L25-27/RConn3 -- Transformer4 132kV / 33kV/RConn3 -- 27/RConn3 -- L27-30/RConn3 -- L27-29/RConn3
  L23-24/LConn1 -- 23/LConn1 -- Load Flow Bus52/LConn1 -- L15-23/RConn1
  L25-26/LConn3 -- 25/RConn3 -- L24-25/RConn3
  L9-10/LConn2 -- 9/LConn2 -- Transformer2 132kV / 33kV/RConn2
  L10-20/RConn1 -- L9-10/RConn1 -- L10-17/RConn1 -- Load Flow Bus54/LConn1 -- 10/RConn1 -- L10-22/LConn1 -- L10-21/LConn1 -- Transformer3 132kV / 33kV/RConn1
  L10-20/RConn2 -- L9-10/RConn2 -- L10-17/RConn2 -- 10/RConn2 -- L10-22/LConn2 -- L10-21/LConn2 -- Transformer3 132kV / 33kV/RConn2
  10/RConn3 -- L10-22/LConn3 -- L10-21/LConn3 -- L10-20/RConn3 -- Transformer3 132kV / 33kV/RConn3 -- L9-10/RConn3 -- L10-17/RConn3
  L6-28/LConn1 -- Transformer2 132kV / 33kV/LConn1 -- 6/LConn1 -- Transformer3 132kV / 33kV/LConn1
  L8-28/RConn2 -- 28/RConn2 -- L6-28/RConn2
  28/RConn3 -- L8-28/RConn3 -- L6-28/RConn3
  L1-2/RConn3 -- L1-3/LConn3 -- 1/LConn3
  L1-2/RConn2 -- 1/LConn2 -- L1-3/LConn2
  L1-2/RConn1 -- 1/LConn1 -- L1-3/LConn1
  Load2/LConn1 -- 2/RConn1 -- Load Flow Bus37/LConn1 -- Gen2/RConn1
  L3-4/LConn2 -- 3/RConn2 -- L1-3/RConn2
  L1-3/RConn3 -- 3/RConn3 -- L3-4/LConn3
  L2-5/RConn2 -- 5/LConn2 -- L5-7/LConn2
  L2-5/RConn3 -- 5/LConn3 -- L5-7/LConn3
  7/LConn1 -- L5-7/RConn1 -- L6-7/LConn1 -- Load Flow Bus42/LConn1
  Transformer3 132kV / 33kV/LConn2 -- L6-28/LConn2 -- Transformer2 132kV / 33kV/LConn2 -- 6/LConn2
  Transformer3 132kV / 33kV/LConn3 -- L6-28/LConn3 -- 6/LConn3 -- Transformer2 132kV / 33kV/LConn3
  28/RConn1 -- L8-28/RConn1 -- L6-28/RConn1
  L12-14/RConn2 -- 14/RConn2 -- L14-15/LConn2
  L14-15/RConn1 -- L12-15/RConn1 -- Load Flow Bus64/LConn1 -- 15/LConn1 -- L15-23/LConn1 -- L15-18/LConn1
  L19-20/RConn2 -- 19/RConn2 -- L18-19/RConn2
  L18-19/LConn2 -- 18/RConn2 -- L15-18/RConn2
  L25-26/LConn1 -- 25/RConn1 -- L24-25/RConn1
  L25-26/LConn2 -- 25/RConn2 -- L24-25/RConn2
  Load8/LConn1 -- Gen4/RConn1 -- 8/LConn1
  Load8/LConn3 -- 8/LConn3 -- Gen4/RConn3
  Load8/LConn2 -- 8/LConn2 -- Gen4/RConn2
  Load5/LConn2 -- 5/RConn2 -- Gen3/RConn2
  Load5/LConn1 -- 5/RConn1 -- Gen3/RConn1
  Load5/LConn3 -- 5/RConn3 -- Gen3/RConn3
  7/RConn1 -- Load7/LConn1
  7/RConn3 -- Load7/LConn3
  7/RConn2 -- Load7/LConn2
  14/LConn3 -- Load14/LConn3
  18/LConn3 -- Load18/LConn3
  30/LConn1 -- Load30/LConn1
  Gen1/RConn1 -- Load Flow Bus28/LConn1 -- 1/RConn1
  Gen1/RConn2 -- 1/RConn2
  Gen1/RConn3 -- 1/RConn3
  Load3/LConn1 -- 3/LConn1
  Load3/LConn2 -- 3/LConn2
  Load3/LConn3 -- 3/LConn3
  L4-6/LConn2 -- L2-4/RConn2 -- 4/RConn2 -- Transformer1 132kV / 33kV/LConn2 -- L3-4/RConn2
  Load Flow Bus63/LConn1 -- L9-11/LConn1 -- 11/LConn1
  L9-11/LConn2 -- 11/LConn2
  L9-11/LConn3 -- 11/LConn3
  11/RConn1 -- Gen5/RConn1
  11/RConn2 -- Gen5/RConn2
  11/RConn3 -- Gen5/RConn3
  13/LConn1 -- Load Flow Bus58/LConn1 -- L12-13/LConn1
  13/LConn3 -- L12-13/LConn3
  Load14/LConn1 -- 14/LConn1
  Load14/LConn2 -- 14/LConn2
  Load18/LConn1 -- 18/LConn1
  Load18/LConn2 -- 18/LConn2
  19/LConn1 -- Load19/LConn1
  19/LConn3 -- Load19/LConn3
  Load19/LConn2 -- 19/LConn2
  L19-20/LConn2 -- 20/LConn2 -- L10-20/LConn2
  21/LConn1 -- Load21/LConn1
  21/LConn2 -- Load21/LConn2
  21/LConn3 -- Load21/LConn3
  22/LConn1 -- L22-24/RConn1
  22/LConn2 -- L22-24/RConn2
  22/LConn3 -- L22-24/RConn3
  26/LConn1 -- Load26/LConn1
  26/LConn2 -- Load26/LConn2
  Load26/LConn3 -- 26/LConn3
  28/LConn1 -- Load Flow Bus45/LConn1 -- Transformer4 132kV / 33kV/LConn1
  Transformer4 132kV / 33kV/LConn3 -- 28/LConn3
  Load29/LConn1 -- 29/LConn1
  Load29/LConn2 -- 29/LConn2
  Load29/LConn3 -- 29/LConn3
  Load30/LConn2 -- 30/LConn2
  Load30/LConn3 -- 30/LConn3
  10/LConn2 -- Load10/LConn2
  10/LConn1 -- Load10/LConn1
  Load10/LConn3 -- 10/LConn3
  L12-14/RConn1 -- Load Flow Bus5/LConn1 -- 14/RConn1 -- L14-15/LConn1
  L12-14/RConn3 -- 14/RConn3 -- L14-15/LConn3
  Load15/LConn1 -- 15/RConn1
  Load15/LConn2 -- 15/RConn2
  Load15/LConn3 -- 15/RConn3
  L14-15/RConn2 -- L12-15/RConn2 -- 15/LConn2 -- L15-18/LConn2 -- L15-23/LConn2
  L15-18/LConn3 -- 15/LConn3 -- L12-15/RConn3 -- L14-15/RConn3 -- L15-23/LConn3
  L18-19/LConn1 -- 18/RConn1 -- Load Flow Bus2/LConn1 -- L15-18/RConn1
  L15-18/RConn3 -- 18/RConn3 -- L18-19/LConn3
  L18-19/RConn1 -- Load Flow Bus7/LConn1 -- 19/RConn1 -- L19-20/RConn1
  L19-20/RConn3 -- 19/RConn3 -- L18-19/RConn3
  L10-20/LConn1 -- 20/LConn1 -- Load Flow Bus62/LConn1 -- L19-20/LConn1
  L10-20/LConn3 -- 20/LConn3 -- L19-20/LConn3
  20/RConn1 -- Load20/LConn1
  20/RConn2 -- Load20/LConn2
  20/RConn3 -- Load20/LConn3
  L21-22/LConn1 -- Load Flow Bus6/LConn1 -- 21/RConn1 -- L10-21/RConn1
  L21-22/LConn2 -- 21/RConn2 -- L10-21/RConn2
  23/RConn2 -- Load23/LConn2
  23/RConn1 -- Load23/LConn1
  Load23/LConn3 -- 23/RConn3
  L15-23/RConn2 -- 23/LConn2 -- L23-24/LConn2
  L15-23/RConn3 -- L23-24/LConn3 -- 23/LConn3
  24/LConn2 -- Load24/LConn2
  24/LConn1 -- Load24/LConn1 -- Load Flow Bus9/LConn1
  24/LConn3 -- Load24/LConn3
  L25-26/RConn3 -- 26/RConn3
  26/RConn1 -- Load Flow Bus8/LConn1 -- L25-26/RConn1
  26/RConn2 -- L25-26/RConn2
  L29-30/RConn1 -- Load Flow Bus11/LConn1 -- 29/RConn1 -- L27-29/LConn1
  L29-30/RConn2 -- 29/RConn2 -- L27-29/LConn2
  L29-30/RConn3 -- 29/RConn3 -- L27-29/LConn3
  L1-3/RConn1 -- Load Flow Bus4/LConn1 -- 3/RConn1 -- L3-4/LConn1
  L29-30/LConn1 -- Load Flow Bus12/LConn1 -- 30/RConn1 -- L27-30/LConn1
  L29-30/LConn2 -- 30/RConn2 -- L27-30/LConn2
  L27-30/LConn3 -- 30/RConn3 -- L29-30/LConn3
  4/LConn1 -- Load4/LConn1
  4/LConn2 -- Load4/LConn2
  4/LConn3 -- Load4/LConn3
  L4-6/LConn1 -- L2-4/RConn1 -- Load Flow Bus3/LConn1 -- 4/RConn1 -- Transformer1 132kV / 33kV/LConn1 -- L3-4/RConn1
  L4-6/LConn3 -- L2-4/RConn3 -- 4/RConn3 -- Transformer1 132kV / 33kV/LConn3 -- L3-4/RConn3
  L5-7/RConn2 -- 7/LConn2 -- L6-7/LConn2
  L6-7/LConn3 -- 7/LConn3 -- L5-7/RConn3
  L2-6/RConn1 -- L6-7/RConn1 -- 6/RConn1 -- L4-6/RConn1 -- Load Flow Bus43/LConn1 -- L6-8/LConn1
  L6-7/RConn2 -- L2-6/RConn2 -- 6/RConn2 -- L4-6/RConn2 -- L6-8/LConn2
  L6-7/RConn3 -- L2-6/RConn3 -- 6/RConn3 -- L6-8/LConn3 -- L4-6/RConn3
  9/RConn1 -- L9-11/RConn1
  9/RConn2 -- L9-11/RConn2
  9/RConn3 -- L9-11/RConn3
  17/RConn1 -- Load17/LConn1
  17/RConn2 -- Load17/LConn2
  17/RConn3 -- Load17/LConn3
  16/RConn1 -- Load16/LConn1
  16/RConn2 -- Load16/LConn2
  16/RConn3 -- Load16/LConn3
  L12-16/RConn2 -- 16/LConn2 -- L16-17/LConn2
  L12-16/RConn3 -- 16/LConn3 -- L16-17/LConn3
  L12-15/LConn2 -- 12/RConn2 -- Transformer1 132kV / 33kV/RConn2 -- L12-16/LConn2 -- L12-13/RConn2 -- L12-14/LConn2
  L2-5/LConn2 -- L2-4/LConn2 -- 2/LConn2 -- L1-2/LConn2 -- L2-6/LConn2
  L1-2/LConn3 -- 2/LConn3 -- L2-4/LConn3 -- L2-6/LConn3 -- L2-5/LConn3
  Load2/LConn3 -- 2/RConn3 -- Gen2/RConn3
  L1-2/LConn1 -- 2/LConn1 -- L2-4/LConn1 -- L2-6/LConn1 -- L2-5/LConn1
  Load2/LConn2 -- 2/RConn2 -- Gen2/RConn2
  L5-7/LConn1 -- Load Flow Bus1/LConn1 -- 5/LConn1 -- L2-5/RConn1
  L8-28/LConn2 -- 8/RConn2 -- L6-8/RConn2
  L8-28/LConn1 -- Load Flow Bus44/LConn1 -- 8/RConn1 -- L6-8/RConn1
  L8-28/LConn3 -- 8/RConn3 -- L6-8/RConn3
  L9-10/LConn1 -- Load Flow Bus53/LConn1 -- 9/LConn1 -- Transformer2 132kV / 33kV/RConn1
  Transformer2 132kV / 33kV/RConn3 -- 9/LConn3 -- L9-10/LConn3
  L12-14/LConn3 -- 12/RConn3 -- Transformer1 132kV / 33kV/RConn3 -- L12-16/LConn3 -- L12-13/RConn3 -- L12-15/LConn3
  L12-14/LConn1 -- L12-15/LConn1 -- Load Flow Bus57/LConn1 -- 12/RConn1 -- Transformer1 132kV / 33kV/RConn1 -- L12-16/LConn1 -- L12-13/RConn1
  12/LConn1 -- Load12/LConn1
  Load12/LConn2 -- 12/LConn2
  12/LConn3 -- Load12/LConn3
  L12-13/LConn2 -- 13/LConn2
  13/RConn1 -- Gen6/RConn1
  Gen6/RConn2 -- 13/RConn2
  Gen6/RConn3 -- 13/RConn3
  L21-22/LConn3 -- 21/RConn3 -- L10-21/RConn3
  L10-17/LConn1 -- Load Flow Bus55/LConn1 -- 17/LConn1 -- L16-17/RConn1
  L10-17/LConn2 -- 17/LConn2 -- L16-17/RConn2
  L10-17/LConn3 -- 17/LConn3 -- L16-17/RConn3
  L12-16/RConn1 -- Load Flow Bus56/LConn1 -- 16/LConn1 -- L16-17/LConn1
  L25-27/LConn1 -- Load Flow Bus10/LConn1 -- 25/LConn1
  25/LConn2 -- L25-27/LConn2
  25/LConn3 -- L25-27/LConn3
  L21-22/RConn2 -- 22/RConn2 -- L10-22/RConn2
  L21-22/RConn3 -- 22/RConn3 -- L10-22/RConn3
  L21-22/RConn1 -- Load Flow Bus13/LConn1 -- 22/RConn1 -- L10-22/RConn1
  28/LConn2 -- Transformer4 132kV / 33kV/LConn2
  L22-24/LConn2 -- 24/RConn2 -- L23-24/RConn2 -- L24-25/LConn2
  L24-25/LConn3 -- L23-24/RConn3 -- 24/RConn3 -- L22-24/LConn3
  L24-25/LConn1 -- 24/RConn1 -- L23-24/RConn1 -- L22-24/LConn1
